simulink model "GesamtAblaufDiagramm_1"  (R2012b)
settings: Solver=FixedStepDiscrete  StartTime=0.0  StopTime=25  RelTol=1e-3
libraries: commutil2 x12, c280xlib x11, c2833xlib x8, idelinklib_tgtpref x2
(part 1 of 2)
settings Model: Creator=mit064  LastModifiedBy=Gelin Wang
settings DataIOCC: SaveOutput=off  SaveTime=off
settings OptimizationCC: OptimizeModelRefInitCode=on  LifeSpan=1
settings HardwareCC: ProdBitPerChar=16  ProdBitPerInt=16  ProdBitPerPointer=16  ProdLargestAtomicInteger=Integer  ProdIntDivRoundTo=Zero  ProdEndianess=LittleEndian  ProdWordSize=16  ProdHWDeviceType=Texas Instruments->C2000
settings RTWCC: SystemTargetFile=idelink_ert.tlc  GenerateMakefile=off  TemplateMakefile=none  Description=IDE Link ERT  ProcessScript=idelink_ert_make_rtw_hook
settings CodeAppCC: IgnoreCustomStorageClasses=off

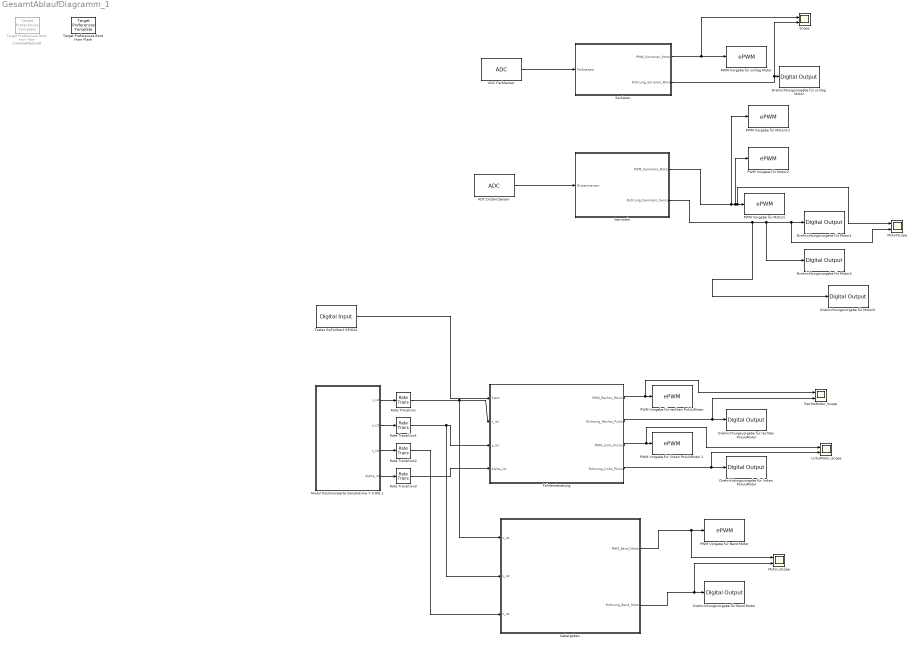
== system GesamtAblaufDiagramm_1 ==
  ADC DistanzSensor : c280xlib/ADC  useModule=A  useMode=Sequential  sourceSOC=Software  sourceSOC1=Software  sourceSOC2=ePWMxB  xint2_ADCSOC=31  Ts=0.001  dType=uint16  postInterrupt=off  numConversionsSingle=1  numConversionsDouble=1  conv0=ADCINA0  conv1=ADCINA1  conv2=ADCINA2  conv3=ADCINA3  conv4=ADCINA4  conv5=ADCINA5  conv6=ADCINA6  conv7=ADCINA7  conv8=ADCINB0  conv9=ADCINB1  conv10=ADCINB2  conv11=ADCINB3  conv12=ADCINB4  conv13=ADCINB5  conv14=ADCINB6  conv15=ADCINB7  convAB0=ADCINA0 and ADCINB0  convAB1=ADCINA1 and ADCINB1  convAB2=ADCINA2 and ADCINB2  convAB3=ADCINA3 and ADCINB3  convAB4=ADCINA4 and ADCINB4  convAB5=ADCINA5 and ADCINB5  convAB6=ADCINA6 and ADCINB6  convAB7=ADCINA7 and ADCINB7  convA0=ADCINA0  convA1=ADCINA1  convA2=ADCINA2  convA3=ADCINA3  convA4=ADCINA4  convA5=ADCINA5  convA6=ADCINA6  convA7=ADCINA7  convB0=ADCINB0  convB1=ADCINB1  convB2=ADCINB2  convB3=ADCINB3  convB4=ADCINB4  convB5=ADCINB5  convB6=ADCINB6  convB7=ADCINB7  c28xmultiPort=off  endma=off  chdma=1
  ADC FarbSensor : c280xlib/ADC  useModule=A  useMode=Sequential  sourceSOC=Software  sourceSOC1=Software  sourceSOC2=ePWMxB  xint2_ADCSOC=31  Ts=0.001  dType=uint16  postInterrupt=off  numConversionsSingle=1  numConversionsDouble=1  conv0=ADCINA0  conv1=ADCINA1  conv2=ADCINA2  conv3=ADCINA3  conv4=ADCINA4  conv5=ADCINA5  conv6=ADCINA6  conv7=ADCINA7  conv8=ADCINB0  conv9=ADCINB1  conv10=ADCINB2  conv11=ADCINB3  conv12=ADCINB4  conv13=ADCINB5  conv14=ADCINB6  conv15=ADCINB7  convAB0=ADCINA0 and ADCINB0  convAB1=ADCINA1 and ADCINB1  convAB2=ADCINA2 and ADCINB2  convAB3=ADCINA3 and ADCINB3  convAB4=ADCINA4 and ADCINB4  convAB5=ADCINA5 and ADCINB5  convAB6=ADCINA6 and ADCINB6  convAB7=ADCINA7 and ADCINB7  convA0=ADCINA0  convA1=ADCINA1  convA2=ADCINA2  convA3=ADCINA3  convA4=ADCINA4  convA5=ADCINA5  convA6=ADCINA6  convA7=ADCINA7  convB0=ADCINB0  convB1=ADCINB1  convB2=ADCINB2  convB3=ADCINB3  convB4=ADCINB4  convB5=ADCINB5  convB6=ADCINB6  convB7=ADCINB7  c28xmultiPort=off  endma=off  chdma=1
  Drehrichtungsvorgabe für Band Motor : c2833xlib/Digital Output  GPIO_Number=GPIO16~GPIO23  GPIO_Bit0=off  GPIO_BIT0_Toggle=off  GPIO_Bit1=off  GPIO_BIT1_Toggle=off  GPIO_Bit2=off  GPIO_BIT2_Toggle=off  GPIO_Bit3=off  GPIO_BIT3_Toggle=off  GPIO_Bit4=off  GPIO_BIT4_Toggle=off  GPIO_Bit5=on  GPIO_BIT5_Toggle=off  GPIO_Bit6=off  GPIO_BIT6_Toggle=off  GPIO_Bit7=off  GPIO_BIT7_Toggle=off
  Drehrichtungsvorgabe für Motor1 : c2833xlib/Digital Output  GPIO_Number=GPIO16~GPIO23  GPIO_Bit0=off  GPIO_BIT0_Toggle=off  GPIO_Bit1=off  GPIO_BIT1_Toggle=off  GPIO_Bit2=off  GPIO_BIT2_Toggle=off  GPIO_Bit3=off  GPIO_BIT3_Toggle=off  GPIO_Bit4=off  GPIO_BIT4_Toggle=off  GPIO_Bit5=on  GPIO_BIT5_Toggle=off  GPIO_Bit6=off  GPIO_BIT6_Toggle=off  GPIO_Bit7=off  GPIO_BIT7_Toggle=off
  Drehrichtungsvorgabe für Motor2 : c2833xlib/Digital Output  GPIO_Number=GPIO16~GPIO23  GPIO_Bit0=off  GPIO_BIT0_Toggle=off  GPIO_Bit1=off  GPIO_BIT1_Toggle=off  GPIO_Bit2=off  GPIO_BIT2_Toggle=off  GPIO_Bit3=off  GPIO_BIT3_Toggle=off  GPIO_Bit4=off  GPIO_BIT4_Toggle=off  GPIO_Bit5=on  GPIO_BIT5_Toggle=off  GPIO_Bit6=off  GPIO_BIT6_Toggle=off  GPIO_Bit7=off  GPIO_BIT7_Toggle=off
  Drehrichtungsvorgabe für Motor3 : c2833xlib/Digital Output  GPIO_Number=GPIO16~GPIO23  GPIO_Bit0=off  GPIO_BIT0_Toggle=off  GPIO_Bit1=off  GPIO_BIT1_Toggle=off  GPIO_Bit2=off  GPIO_BIT2_Toggle=off  GPIO_Bit3=off  GPIO_BIT3_Toggle=off  GPIO_Bit4=off  GPIO_BIT4_Toggle=off  GPIO_Bit5=on  GPIO_BIT5_Toggle=off  GPIO_Bit6=off  GPIO_BIT6_Toggle=off  GPIO_Bit7=off  GPIO_BIT7_Toggle=off
  Drehrichtungsvorgabe für linken PoluluMotor : c2833xlib/Digital Output  GPIO_Number=GPIO16~GPIO23  GPIO_Bit0=off  GPIO_BIT0_Toggle=off  GPIO_Bit1=off  GPIO_BIT1_Toggle=off  GPIO_Bit2=off  GPIO_BIT2_Toggle=off  GPIO_Bit3=off  GPIO_BIT3_Toggle=off  GPIO_Bit4=off  GPIO_BIT4_Toggle=off  GPIO_Bit5=on  GPIO_BIT5_Toggle=off  GPIO_Bit6=off  GPIO_BIT6_Toggle=off  GPIO_Bit7=off  GPIO_BIT7_Toggle=off
  Drehrichtungsvorgabe für rechten PoluluMotor : c2833xlib/Digital Output  GPIO_Number=GPIO16~GPIO23  GPIO_Bit0=off  GPIO_BIT0_Toggle=off  GPIO_Bit1=off  GPIO_BIT1_Toggle=off  GPIO_Bit2=off  GPIO_BIT2_Toggle=off  GPIO_Bit3=off  GPIO_BIT3_Toggle=off  GPIO_Bit4=off  GPIO_BIT4_Toggle=off  GPIO_Bit5=on  GPIO_BIT5_Toggle=off  GPIO_Bit6=off  GPIO_BIT6_Toggle=off  GPIO_Bit7=off  GPIO_BIT7_Toggle=off
  Drehrichtungsvorgabe für schlag Motor : c2833xlib/Digital Output  GPIO_Number=GPIO16~GPIO23  GPIO_Bit0=off  GPIO_BIT0_Toggle=off  GPIO_Bit1=off  GPIO_BIT1_Toggle=off  GPIO_Bit2=off  GPIO_BIT2_Toggle=off  GPIO_Bit3=off  GPIO_BIT3_Toggle=off  GPIO_Bit4=off  GPIO_BIT4_Toggle=off  GPIO_Bit5=on  GPIO_BIT5_Toggle=off  GPIO_Bit6=off  GPIO_BIT6_Toggle=off  GPIO_Bit7=off  GPIO_BIT7_Toggle=off
  "Fahransteuerung " : Subsystem
  LinksMotor_Scope : Scope  NumInputPorts=2
      settings: YMin=-5~-5  YMax=5~5  SaveName=ScopeData3
  Modul Positionswerte Sampletime = 0.001 s : Subsystem
  MotorScope : Scope  NumInputPorts=2
      settings: YMin=-5~-5  YMax=100~5  SaveName=ScopeData4
  Motor_Scope : Scope  NumInputPorts=2
      settings: YMin=-5~-5  YMax=5~5
  "PWM Vorgabe für Band Motor " : c280xlib/ePWM  checkMode=off  useModule=ePWM2  periodUnits=Clock cycles  timerSource=Specify via dialog  timerPeriod_clk=64000  timerPeriod_sec=0.0001  countingMode=Up  synchronizationOption=Disable  synchronizationEnable=off  phaseActiveEnable=Disable  phaseDirection=Count down after sync  phaseActive=0  clockPrescale=1  HSclockPrescale=1  ePWMxAStatus=off  CMPAUnits=Clock cycles  CMPASource=Specify via dialog  CMPAValue_per=50  CMPAValue_clk=32000  ePWMxAactionLogic1=Do nothing  ePWMxAactionLogic2=Clear  ePWMxAactionLogic3=Set  ePWMxAactionLogic4=Do nothing  ePWMxAactionLogic5=Do nothing  ePWMxAactionLogic6=Do nothing  ePWMxALoadMode=Load on CTR=Zero  ePWMxACSFenable=off  ePWMxACSFvalue=Forcing Disable  ePWMxASFreload=Zero  enHRPWM=off  HRPWM_LoadMode=CTR=ZERO  HRPWM_CTLMode=Phase control mode  HRPWM_EDGMode=Both edge  enSFO=on  ePWMxBStatus=on  CMPBUnits=Percentages  CMPBSource=Input port  CMPBValue_per=0  CMPBValue_clk=32000  ePWMxBactionLogic1=Do nothing  ePWMxBactionLogic2=Set  ePWMxBactionLogic3=Do nothing  ePWMxBactionLogic4=Do nothing  ePWMxBactionLogic5=Clear  ePWMxBactionLogic6=Do nothing  ePWMxBLoadMode=Load on CTR=Zero  ePWMxBCSFenable=off  ePWMxBCSFvalue=Forcing Disable  ePWMxBSFreload=Zero  enableDBePWMxA=off  enableDBePWMxB=off  DBpolarity=AH  DBedgeDelay=Positive  DBSource_ePWMxA=ePWMxA  DBSource_ePWMxB=ePWMxA  DBperiodSource=Specify via dialog  REDperiod=0  FEDperiod=0  adcstartModuleA=off  adcrequestEventA=First event  adcstartEventA=CTR=Zero  adcstartModuleB=off  adcrequestEventB=First event  adcstartEventB=CTR=Zero  intEn=off  intPrd=First event  intSel=CTR=Zero  chopperEnable=off  chopperFrequency=1  chopperFirstwidth=1  chopperDuty=12.5%  tripZonesource=Specify via dialog  tzselOSHT1=off  tzselOSHT2=off  tzselOSHT3=off  tzselOSHT4=off  tzselOSHT5=off  tzselOSHT6=off  tzselCBC1=off  tzselCBC2=off  tzselCBC3=off  tzselCBC4=off  tzselCBC5=off  tzselCBC6=off  enTzOstIntr=off  enTzCbcIntr=off  ePWMxAforced=No action  ePWMxBforced=No action  timerPeriod=-1  ePWMxAValue=0  ePWMxBValue=0  tripZoneoption=OSHT
  "PWM Vorgabe für Motor1 " : c280xlib/ePWM  checkMode=off  useModule=ePWM2  periodUnits=Clock cycles  timerSource=Specify via dialog  timerPeriod_clk=64000  timerPeriod_sec=0.0001  countingMode=Up  synchronizationOption=Disable  synchronizationEnable=off  phaseActiveEnable=Disable  phaseDirection=Count down after sync  phaseActive=0  clockPrescale=1  HSclockPrescale=1  ePWMxAStatus=off  CMPAUnits=Clock cycles  CMPASource=Specify via dialog  CMPAValue_per=50  CMPAValue_clk=32000  ePWMxAactionLogic1=Do nothing  ePWMxAactionLogic2=Clear  ePWMxAactionLogic3=Set  ePWMxAactionLogic4=Do nothing  ePWMxAactionLogic5=Do nothing  ePWMxAactionLogic6=Do nothing  ePWMxALoadMode=Load on CTR=Zero  ePWMxACSFenable=off  ePWMxACSFvalue=Forcing Disable  ePWMxASFreload=Zero  enHRPWM=off  HRPWM_LoadMode=CTR=ZERO  HRPWM_CTLMode=Phase control mode  HRPWM_EDGMode=Both edge  enSFO=on  ePWMxBStatus=on  CMPBUnits=Percentages  CMPBSource=Input port  CMPBValue_per=0  CMPBValue_clk=32000  ePWMxBactionLogic1=Do nothing  ePWMxBactionLogic2=Set  ePWMxBactionLogic3=Do nothing  ePWMxBactionLogic4=Do nothing  ePWMxBactionLogic5=Clear  ePWMxBactionLogic6=Do nothing  ePWMxBLoadMode=Load on CTR=Zero  ePWMxBCSFenable=off  ePWMxBCSFvalue=Forcing Disable  ePWMxBSFreload=Zero  enableDBePWMxA=off  enableDBePWMxB=off  DBpolarity=AH  DBedgeDelay=Positive  DBSource_ePWMxA=ePWMxA  DBSource_ePWMxB=ePWMxA  DBperiodSource=Specify via dialog  REDperiod=0  FEDperiod=0  adcstartModuleA=off  adcrequestEventA=First event  adcstartEventA=CTR=Zero  adcstartModuleB=off  adcrequestEventB=First event  adcstartEventB=CTR=Zero  intEn=off  intPrd=First event  intSel=CTR=Zero  chopperEnable=off  chopperFrequency=1  chopperFirstwidth=1  chopperDuty=12.5%  tripZonesource=Specify via dialog  tzselOSHT1=off  tzselOSHT2=off  tzselOSHT3=off  tzselOSHT4=off  tzselOSHT5=off  tzselOSHT6=off  tzselCBC1=off  tzselCBC2=off  tzselCBC3=off  tzselCBC4=off  tzselCBC5=off  tzselCBC6=off  enTzOstIntr=off  enTzCbcIntr=off  ePWMxAforced=No action  ePWMxBforced=No action  timerPeriod=-1  ePWMxAValue=0  ePWMxBValue=0  tripZoneoption=OSHT
  "PWM Vorgabe für Motor2 " : c280xlib/ePWM  checkMode=off  useModule=ePWM2  periodUnits=Clock cycles  timerSource=Specify via dialog  timerPeriod_clk=64000  timerPeriod_sec=0.0001  countingMode=Up  synchronizationOption=Disable  synchronizationEnable=off  phaseActiveEnable=Disable  phaseDirection=Count down after sync  phaseActive=0  clockPrescale=1  HSclockPrescale=1  ePWMxAStatus=off  CMPAUnits=Clock cycles  CMPASource=Specify via dialog  CMPAValue_per=50  CMPAValue_clk=32000  ePWMxAactionLogic1=Do nothing  ePWMxAactionLogic2=Clear  ePWMxAactionLogic3=Set  ePWMxAactionLogic4=Do nothing  ePWMxAactionLogic5=Do nothing  ePWMxAactionLogic6=Do nothing  ePWMxALoadMode=Load on CTR=Zero  ePWMxACSFenable=off  ePWMxACSFvalue=Forcing Disable  ePWMxASFreload=Zero  enHRPWM=off  HRPWM_LoadMode=CTR=ZERO  HRPWM_CTLMode=Phase control mode  HRPWM_EDGMode=Both edge  enSFO=on  ePWMxBStatus=on  CMPBUnits=Percentages  CMPBSource=Input port  CMPBValue_per=0  CMPBValue_clk=32000  ePWMxBactionLogic1=Do nothing  ePWMxBactionLogic2=Set  ePWMxBactionLogic3=Do nothing  ePWMxBactionLogic4=Do nothing  ePWMxBactionLogic5=Clear  ePWMxBactionLogic6=Do nothing  ePWMxBLoadMode=Load on CTR=Zero  ePWMxBCSFenable=off  ePWMxBCSFvalue=Forcing Disable  ePWMxBSFreload=Zero  enableDBePWMxA=off  enableDBePWMxB=off  DBpolarity=AH  DBedgeDelay=Positive  DBSource_ePWMxA=ePWMxA  DBSource_ePWMxB=ePWMxA  DBperiodSource=Specify via dialog  REDperiod=0  FEDperiod=0  adcstartModuleA=off  adcrequestEventA=First event  adcstartEventA=CTR=Zero  adcstartModuleB=off  adcrequestEventB=First event  adcstartEventB=CTR=Zero  intEn=off  intPrd=First event  intSel=CTR=Zero  chopperEnable=off  chopperFrequency=1  chopperFirstwidth=1  chopperDuty=12.5%  tripZonesource=Specify via dialog  tzselOSHT1=off  tzselOSHT2=off  tzselOSHT3=off  tzselOSHT4=off  tzselOSHT5=off  tzselOSHT6=off  tzselCBC1=off  tzselCBC2=off  tzselCBC3=off  tzselCBC4=off  tzselCBC5=off  tzselCBC6=off  enTzOstIntr=off  enTzCbcIntr=off  ePWMxAforced=No action  ePWMxBforced=No action  timerPeriod=-1  ePWMxAValue=0  ePWMxBValue=0  tripZoneoption=OSHT
  PWM Vorgabe für Motor3 2 : c280xlib/ePWM  checkMode=off  useModule=ePWM2  periodUnits=Clock cycles  timerSource=Specify via dialog  timerPeriod_clk=64000  timerPeriod_sec=0.0001  countingMode=Up  synchronizationOption=Disable  synchronizationEnable=off  phaseActiveEnable=Disable  phaseDirection=Count down after sync  phaseActive=0  clockPrescale=1  HSclockPrescale=1  ePWMxAStatus=off  CMPAUnits=Clock cycles  CMPASource=Specify via dialog  CMPAValue_per=50  CMPAValue_clk=32000  ePWMxAactionLogic1=Do nothing  ePWMxAactionLogic2=Clear  ePWMxAactionLogic3=Set  ePWMxAactionLogic4=Do nothing  ePWMxAactionLogic5=Do nothing  ePWMxAactionLogic6=Do nothing  ePWMxALoadMode=Load on CTR=Zero  ePWMxACSFenable=off  ePWMxACSFvalue=Forcing Disable  ePWMxASFreload=Zero  enHRPWM=off  HRPWM_LoadMode=CTR=ZERO  HRPWM_CTLMode=Phase control mode  HRPWM_EDGMode=Both edge  enSFO=on  ePWMxBStatus=on  CMPBUnits=Percentages  CMPBSource=Input port  CMPBValue_per=0  CMPBValue_clk=32000  ePWMxBactionLogic1=Do nothing  ePWMxBactionLogic2=Set  ePWMxBactionLogic3=Do nothing  ePWMxBactionLogic4=Do nothing  ePWMxBactionLogic5=Clear  ePWMxBactionLogic6=Do nothing  ePWMxBLoadMode=Load on CTR=Zero  ePWMxBCSFenable=off  ePWMxBCSFvalue=Forcing Disable  ePWMxBSFreload=Zero  enableDBePWMxA=off  enableDBePWMxB=off  DBpolarity=AH  DBedgeDelay=Positive  DBSource_ePWMxA=ePWMxA  DBSource_ePWMxB=ePWMxA  DBperiodSource=Specify via dialog  REDperiod=0  FEDperiod=0  adcstartModuleA=off  adcrequestEventA=First event  adcstartEventA=CTR=Zero  adcstartModuleB=off  adcrequestEventB=First event  adcstartEventB=CTR=Zero  intEn=off  intPrd=First event  intSel=CTR=Zero  chopperEnable=off  chopperFrequency=1  chopperFirstwidth=1  chopperDuty=12.5%  tripZonesource=Specify via dialog  tzselOSHT1=off  tzselOSHT2=off  tzselOSHT3=off  tzselOSHT4=off  tzselOSHT5=off  tzselOSHT6=off  tzselCBC1=off  tzselCBC2=off  tzselCBC3=off  tzselCBC4=off  tzselCBC5=off  tzselCBC6=off  enTzOstIntr=off  enTzCbcIntr=off  ePWMxAforced=No action  ePWMxBforced=No action  timerPeriod=-1  ePWMxAValue=0  ePWMxBValue=0  tripZoneoption=OSHT
  PWM Vorgabe für linken PoluluMotor 1 : c280xlib/ePWM  checkMode=off  useModule=ePWM2  periodUnits=Clock cycles  timerSource=Specify via dialog  timerPeriod_clk=64000  timerPeriod_sec=0.0001  countingMode=Up  synchronizationOption=Disable  synchronizationEnable=off  phaseActiveEnable=Disable  phaseDirection=Count down after sync  phaseActive=0  clockPrescale=1  HSclockPrescale=1  ePWMxAStatus=off  CMPAUnits=Clock cycles  CMPASource=Specify via dialog  CMPAValue_per=50  CMPAValue_clk=32000  ePWMxAactionLogic1=Do nothing  ePWMxAactionLogic2=Clear  ePWMxAactionLogic3=Set  ePWMxAactionLogic4=Do nothing  ePWMxAactionLogic5=Do nothing  ePWMxAactionLogic6=Do nothing  ePWMxALoadMode=Load on CTR=Zero  ePWMxACSFenable=off  ePWMxACSFvalue=Forcing Disable  ePWMxASFreload=Zero  enHRPWM=off  HRPWM_LoadMode=CTR=ZERO  HRPWM_CTLMode=Phase control mode  HRPWM_EDGMode=Both edge  enSFO=on  ePWMxBStatus=on  CMPBUnits=Percentages  CMPBSource=Input port  CMPBValue_per=0  CMPBValue_clk=32000  ePWMxBactionLogic1=Do nothing  ePWMxBactionLogic2=Set  ePWMxBactionLogic3=Do nothing  ePWMxBactionLogic4=Do nothing  ePWMxBactionLogic5=Clear  ePWMxBactionLogic6=Do nothing  ePWMxBLoadMode=Load on CTR=Zero  ePWMxBCSFenable=off  ePWMxBCSFvalue=Forcing Disable  ePWMxBSFreload=Zero  enableDBePWMxA=off  enableDBePWMxB=off  DBpolarity=AH  DBedgeDelay=Positive  DBSource_ePWMxA=ePWMxA  DBSource_ePWMxB=ePWMxA  DBperiodSource=Specify via dialog  REDperiod=0  FEDperiod=0  adcstartModuleA=off  adcrequestEventA=First event  adcstartEventA=CTR=Zero  adcstartModuleB=off  adcrequestEventB=First event  adcstartEventB=CTR=Zero  intEn=off  intPrd=First event  intSel=CTR=Zero  chopperEnable=off  chopperFrequency=1  chopperFirstwidth=1  chopperDuty=12.5%  tripZonesource=Specify via dialog  tzselOSHT1=off  tzselOSHT2=off  tzselOSHT3=off  tzselOSHT4=off  tzselOSHT5=off  tzselOSHT6=off  tzselCBC1=off  tzselCBC2=off  tzselCBC3=off  tzselCBC4=off  tzselCBC5=off  tzselCBC6=off  enTzOstIntr=off  enTzCbcIntr=off  ePWMxAforced=No action  ePWMxBforced=No action  timerPeriod=-1  ePWMxAValue=0  ePWMxBValue=0  tripZoneoption=OSHT
  "PWM Vorgabe für rechten PoluluMotor " : c280xlib/ePWM  checkMode=off  useModule=ePWM2  periodUnits=Clock cycles  timerSource=Specify via dialog  timerPeriod_clk=64000  timerPeriod_sec=0.0001  countingMode=Up  synchronizationOption=Disable  synchronizationEnable=off  phaseActiveEnable=Disable  phaseDirection=Count down after sync  phaseActive=0  clockPrescale=1  HSclockPrescale=1  ePWMxAStatus=off  CMPAUnits=Clock cycles  CMPASource=Specify via dialog  CMPAValue_per=50  CMPAValue_clk=32000  ePWMxAactionLogic1=Do nothing  ePWMxAactionLogic2=Clear  ePWMxAactionLogic3=Set  ePWMxAactionLogic4=Do nothing  ePWMxAactionLogic5=Do nothing  ePWMxAactionLogic6=Do nothing  ePWMxALoadMode=Load on CTR=Zero  ePWMxACSFenable=off  ePWMxACSFvalue=Forcing Disable  ePWMxASFreload=Zero  enHRPWM=off  HRPWM_LoadMode=CTR=ZERO  HRPWM_CTLMode=Phase control mode  HRPWM_EDGMode=Both edge  enSFO=on  ePWMxBStatus=on  CMPBUnits=Percentages  CMPBSource=Input port  CMPBValue_per=0  CMPBValue_clk=32000  ePWMxBactionLogic1=Do nothing  ePWMxBactionLogic2=Set  ePWMxBactionLogic3=Do nothing  ePWMxBactionLogic4=Do nothing  ePWMxBactionLogic5=Clear  ePWMxBactionLogic6=Do nothing  ePWMxBLoadMode=Load on CTR=Zero  ePWMxBCSFenable=off  ePWMxBCSFvalue=Forcing Disable  ePWMxBSFreload=Zero  enableDBePWMxA=off  enableDBePWMxB=off  DBpolarity=AH  DBedgeDelay=Positive  DBSource_ePWMxA=ePWMxA  DBSource_ePWMxB=ePWMxA  DBperiodSource=Specify via dialog  REDperiod=0  FEDperiod=0  adcstartModuleA=off  adcrequestEventA=First event  adcstartEventA=CTR=Zero  adcstartModuleB=off  adcrequestEventB=First event  adcstartEventB=CTR=Zero  intEn=off  intPrd=First event  intSel=CTR=Zero  chopperEnable=off  chopperFrequency=1  chopperFirstwidth=1  chopperDuty=12.5%  tripZonesource=Specify via dialog  tzselOSHT1=off  tzselOSHT2=off  tzselOSHT3=off  tzselOSHT4=off  tzselOSHT5=off  tzselOSHT6=off  tzselCBC1=off  tzselCBC2=off  tzselCBC3=off  tzselCBC4=off  tzselCBC5=off  tzselCBC6=off  enTzOstIntr=off  enTzCbcIntr=off  ePWMxAforced=No action  ePWMxBforced=No action  timerPeriod=-1  ePWMxAValue=0  ePWMxBValue=0  tripZoneoption=OSHT
  "PWM Vorgabe für schlag Motor " : c280xlib/ePWM  checkMode=off  useModule=ePWM2  periodUnits=Clock cycles  timerSource=Specify via dialog  timerPeriod_clk=64000  timerPeriod_sec=0.0001  countingMode=Up  synchronizationOption=Disable  synchronizationEnable=off  phaseActiveEnable=Disable  phaseDirection=Count down after sync  phaseActive=0  clockPrescale=1  HSclockPrescale=1  ePWMxAStatus=off  CMPAUnits=Clock cycles  CMPASource=Specify via dialog  CMPAValue_per=50  CMPAValue_clk=32000  ePWMxAactionLogic1=Do nothing  ePWMxAactionLogic2=Clear  ePWMxAactionLogic3=Set  ePWMxAactionLogic4=Do nothing  ePWMxAactionLogic5=Do nothing  ePWMxAactionLogic6=Do nothing  ePWMxALoadMode=Load on CTR=Zero  ePWMxACSFenable=off  ePWMxACSFvalue=Forcing Disable  ePWMxASFreload=Zero  enHRPWM=off  HRPWM_LoadMode=CTR=ZERO  HRPWM_CTLMode=Phase control mode  HRPWM_EDGMode=Both edge  enSFO=on  ePWMxBStatus=on  CMPBUnits=Percentages  CMPBSource=Input port  CMPBValue_per=0  CMPBValue_clk=32000  ePWMxBactionLogic1=Do nothing  ePWMxBactionLogic2=Set  ePWMxBactionLogic3=Do nothing  ePWMxBactionLogic4=Do nothing  ePWMxBactionLogic5=Clear  ePWMxBactionLogic6=Do nothing  ePWMxBLoadMode=Load on CTR=Zero  ePWMxBCSFenable=off  ePWMxBCSFvalue=Forcing Disable  ePWMxBSFreload=Zero  enableDBePWMxA=off  enableDBePWMxB=off  DBpolarity=AH  DBedgeDelay=Positive  DBSource_ePWMxA=ePWMxA  DBSource_ePWMxB=ePWMxA  DBperiodSource=Specify via dialog  REDperiod=0  FEDperiod=0  adcstartModuleA=off  adcrequestEventA=First event  adcstartEventA=CTR=Zero  adcstartModuleB=off  adcrequestEventB=First event  adcstartEventB=CTR=Zero  intEn=off  intPrd=First event  intSel=CTR=Zero  chopperEnable=off  chopperFrequency=1  chopperFirstwidth=1  chopperDuty=12.5%  tripZonesource=Specify via dialog  tzselOSHT1=off  tzselOSHT2=off  tzselOSHT3=off  tzselOSHT4=off  tzselOSHT5=off  tzselOSHT6=off  tzselCBC1=off  tzselCBC2=off  tzselCBC3=off  tzselCBC4=off  tzselCBC5=off  tzselCBC6=off  enTzOstIntr=off  enTzCbcIntr=off  ePWMxAforced=No action  ePWMxBforced=No action  timerPeriod=-1  ePWMxAValue=0  ePWMxBValue=0  tripZoneoption=OSHT
  Rate Transition{,1..3} (4 alike) : RateTransition  OutPortSampleTime=0.01
  RechtsMotor_Scope : Scope  NumInputPorts=2
      settings: YMin=-5~-5  YMax=5~5  SaveName=ScopeData2
  Sammeln : Subsystem
  Scope : Scope  NumInputPorts=2
      settings: YMin=-5~-5  YMax=5~5
  Sortieren : Subsystem
  Target Preferences Boot from Flash : idelinklib_tgtpref/Target Preferences Template  Tag=ccslinktgtpref_ccsv4  library=off
  Target Preferences Boot from Ram : idelinklib_tgtpref/Target Preferences Template  Tag=ccslinktgtpref_ccsv4  Commented=on  library=off
  Taster GoForStart GPIO24 : c2833xlib/Digital Input  GPIO_Number=GPIO24~GPIO31  GPIO_Bit0=on  GPIO_Bit1=off  GPIO_Bit2=off  GPIO_Bit3=off  GPIO_Bit4=off  GPIO_Bit5=off  GPIO_Bit6=off  GPIO_Bit7=off  sampleTime=0.001  dataType=auto  GPIO_Bit0_Qualification=Sync to SYSCLKOUT  GPIO_Bit1_Qualification=Sync to SYSCLKOUT  GPIO_Bit2_Qualification=Sync to SYSCLKOUT  GPIO_Bit3_Qualification=Sync to SYSCLKOUT  GPIO_Bit4_Qualification=Sync to SYSCLKOUT  GPIO_Bit5_Qualification=Sync to SYSCLKOUT  GPIO_Bit6_Qualification=Sync to SYSCLKOUT  GPIO_Bit7_Qualification=Sync to SYSCLKOUT  Qualification_Period=-1
  Uebergeben : Subsystem
  wires:
  Modul Positionswerte Sampletime = 0.001 s/1(x_ist) -> Rate Transition/1
  Modul Positionswerte Sampletime = 0.001 s/4(alpha_ist) -> Rate Transition3/1
  Modul Positionswerte Sampletime = 0.001 s/3(z_ist) -> Rate Transition2/1
  Modul Positionswerte Sampletime = 0.001 s/2(y_ist) -> Rate Transition1/1
  Rate Transition/1 -> Uebergeben/1(x_ist), "Fahransteuerung "/2(x_ist)
  Rate Transition1/1 -> Uebergeben/2(y_ist), "Fahransteuerung "/3(y_ist)
  Rate Transition3/1 -> "Fahransteuerung "/4(alpha_ist)
  "Fahransteuerung "/1(PWM_Rechts_Polulu) -> RechtsMotor_Scope/1, "PWM Vorgabe für rechten PoluluMotor "/1
  "Fahransteuerung "/2(Richtung_Rechts_Pulolo) -> RechtsMotor_Scope/2, Drehrichtungsvorgabe für rechten PoluluMotor/1
  "Fahransteuerung "/3(PWM_Links_Polulu) -> LinksMotor_Scope/1, PWM Vorgabe für linken PoluluMotor 1/1
  "Fahransteuerung "/4(Richtung_Links_Polulu) -> LinksMotor_Scope/2, Drehrichtungsvorgabe für linken PoluluMotor/1
  Rate Transition2/1 -> Uebergeben/3(z_ist)
  Uebergeben/1(PWM_Band_Motor) -> Motor_Scope/1, "PWM Vorgabe für Band Motor "/1
  Uebergeben/2(Richtung_Band_Motor) -> Motor_Scope/2, Drehrichtungsvorgabe für Band Motor/1
  ADC DistanzSensor/1 -> Sammeln/1(Distanzsensor)
  ADC FarbSensor/1 -> Sortieren/1(Farbsensor)
  Sortieren/2(Richtung_Sorieren_Motor) -> Scope/2, Drehrichtungsvorgabe für schlag Motor/1
  Sortieren/1(PMW_Sortieren_Motor) -> Scope/1, "PWM Vorgabe für schlag Motor "/1
  Sammeln/2(Richtung_Sammeln_Sensor) -> Drehrichtungsvorgabe für Motor3/1, Drehrichtungsvorgabe für Motor2/1, MotorScope/2, Drehrichtungsvorgabe für Motor1/1
  Sammeln/1(PWM_Sammeln_Motor) -> PWM Vorgabe für Motor3 2/1, "PWM Vorgabe für Motor2 "/1, MotorScope/1, "PWM Vorgabe für Motor1 "/1
  Taster GoForStart GPIO24/1 -> "Fahransteuerung "/1(Start)

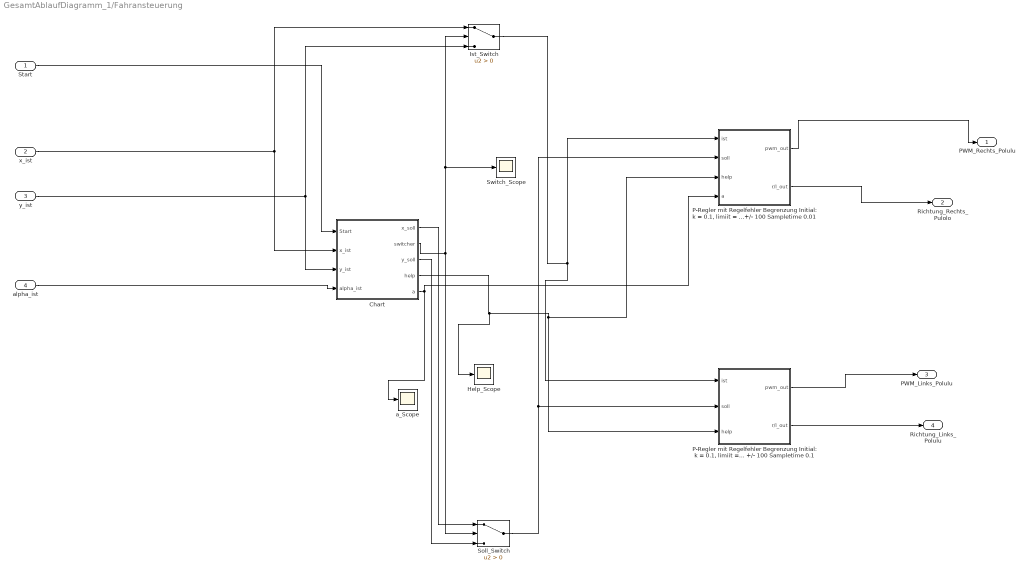
== system GesamtAblaufDiagramm_1/Fahransteuerung  ==
  Start : Inport
  x_ist : Inport  Port=2
  y_ist : Inport  Port=3
  alpha_ist : Inport  Port=4
  Chart : Stateflow chart  TreatAsAtomicUnit=on
  Help_Scope : Scope
      settings: SaveName=ScopeData5
  Ist_Switch : Switch  Criteria=u2 > Threshold
  "P-Regler mit Regelfehler Begrenzung Initial: k = 0.1, limiit = +/- 100 Sampletime 0.01" : Subsystem
  "P-Regler mit Regelfehler Begrenzung Initial: k = 0.1, limiit = +/- 100 Sampletime 0.1" : Subsystem
  Soll_Switch : Switch  Criteria=u2 > Threshold
  Switch_Scope : Scope
      settings: SaveName=ScopeData6
  a_Scope : Scope
      settings: SaveName=ScopeData7
  PWM_Rechts_Polulu : Outport
  Richtung_Rechts_Pulolo : Outport  Port=2
  PWM_Links_Polulu : Outport  Port=3
  Richtung_Links_Polulu : Outport  Port=4
  wires:
  "P-Regler mit Regelfehler Begrenzung Initial: k = 0.1, limiit = +/- 100 Sampletime 0.01"/2(r/l_out) -> Richtung_Rechts_Pulolo/1
  "P-Regler mit Regelfehler Begrenzung Initial: k = 0.1, limiit = +/- 100 Sampletime 0.01"/1(pwm_out) -> PWM_Rechts_Polulu/1
  Ist_Switch/1 -> "P-Regler mit Regelfehler Begrenzung Initial: k = 0.1, limiit = +/- 100 Sampletime 0.1"/1(ist), "P-Regler mit Regelfehler Begrenzung Initial: k = 0.1, limiit = +/- 100 Sampletime 0.01"/1(ist)
  Soll_Switch/1 -> "P-Regler mit Regelfehler Begrenzung Initial: k = 0.1, limiit = +/- 100 Sampletime 0.01"/2(soll), "P-Regler mit Regelfehler Begrenzung Initial: k = 0.1, limiit = +/- 100 Sampletime 0.1"/2(soll)
  Chart/2(switcher) -> Soll_Switch/2, Switch_Scope/1, Ist_Switch/2
  Chart/1(x_soll) -> Soll_Switch/1
  Chart/3(y_soll) -> Soll_Switch/3
  Chart/4(help) -> Help_Scope/1, "P-Regler mit Regelfehler Begrenzung Initial: k = 0.1, limiit = +/- 100 Sampletime 0.01"/3(help), "P-Regler mit Regelfehler Begrenzung Initial: k = 0.1, limiit = +/- 100 Sampletime 0.1"/3(help)
  x_ist/1 -> Chart/2(x_ist), Ist_Switch/1
  y_ist/1 -> Chart/3(y_ist), Ist_Switch/3
  alpha_ist/1 -> Chart/4(alpha_ist)
  "P-Regler mit Regelfehler Begrenzung Initial: k = 0.1, limiit = +/- 100 Sampletime 0.1"/1(pwm_out) -> PWM_Links_Polulu/1
  "P-Regler mit Regelfehler Begrenzung Initial: k = 0.1, limiit = +/- 100 Sampletime 0.1"/2(r/l_out) -> Richtung_Links_Polulu/1
  Chart/5(a) -> a_Scope/1, "P-Regler mit Regelfehler Begrenzung Initial: k = 0.1, limiit = +/- 100 Sampletime 0.01"/4(a)
  Start/1 -> Chart/1(Start)

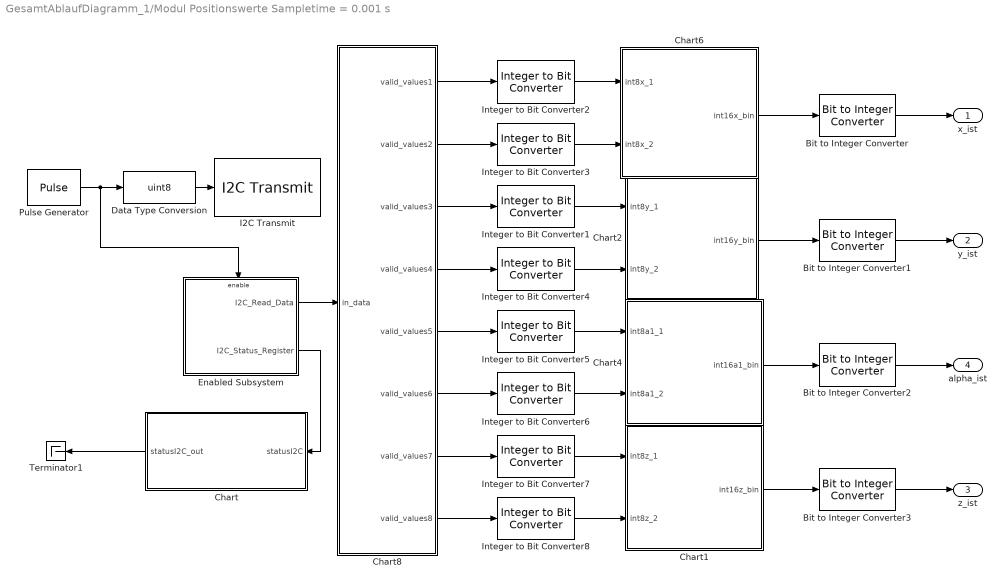
== system GesamtAblaufDiagramm_1/Modul Positionswerte Sampletime = 0.001 s ==
  Bit to Integer Converter{,1..3} (4 alike) : commutil2/Bit to Integer Converter  nbits=16  bitOrder=MSB first  signedOutputValues=Signed  outDtype=Inherit via internal rule  outDtypeSigned=Inherit via internal rule
  Chart : Stateflow chart  TreatAsAtomicUnit=on
  Chart1 : Stateflow chart  TreatAsAtomicUnit=on
  Chart2 : Stateflow chart  TreatAsAtomicUnit=on
  Chart4 : Stateflow chart  TreatAsAtomicUnit=on
  Chart6 : Stateflow chart  TreatAsAtomicUnit=on
  Chart8 : Stateflow chart  TreatAsAtomicUnit=on
  Data Type Conversion : DataTypeConversion  OutDataTypeStr=uint8
  Enabled Subsystem : Subsystem  TreatAsAtomicUnit=on
  I2C Transmit : c280xlib/I2C Transmit  addrFormat=7-Bit addressing  saSource=Specify via dialog  SAR=80  bitCount=8  STP=off  RM=off  STR=off
  Integer to Bit Converter{1..8} (8 alike) : commutil2/Integer to Bit Converter  nbits=8  signedInputValues=Unsigned  bitOrder=MSB first  outDtype=uint8
  Pulse Generator : DiscretePulseGenerator  Period=250  PulseWidth=249  SampleTime=0.001
  Terminator1 : Terminator
  x_ist : Outport
  y_ist : Outport  Port=2
  z_ist : Outport  Port=3
  alpha_ist : Outport  Port=4
  wires:
  Chart8/5(valid_values5) -> Integer to Bit Converter5/1
  Chart8/2(valid_values2) -> Integer to Bit Converter3/1
  Chart8/4(valid_values4) -> Integer to Bit Converter4/1
  Chart2/1(int16y_bin) -> Bit to Integer Converter1/1
  Chart8/1(valid_values1) -> Integer to Bit Converter2/1
  Chart8/3(valid_values3) -> Integer to Bit Converter1/1
  Integer to Bit Converter3/1 -> Chart6/2(int8x_2)
  Chart6/1(int16x_bin) -> Bit to Integer Converter/1
  Integer to Bit Converter1/1 -> Chart2/1(int8y_1)
  Integer to Bit Converter2/1 -> Chart6/1(int8x_1)
  Integer to Bit Converter4/1 -> Chart2/2(int8y_2)
  Bit to Integer Converter1/1 -> y_ist/1
  Integer to Bit Converter5/1 -> Chart4/1(int8a1_1)
  Integer to Bit Converter6/1 -> Chart4/2(int8a1_2)
  Bit to Integer Converter/1 -> x_ist/1
  Bit to Integer Converter2/1 -> alpha_ist/1
  Chart8/6(valid_values6) -> Integer to Bit Converter6/1
  Chart4/1(int16a1_bin) -> Bit to Integer Converter2/1
  Chart1/1(int16z_bin) -> Bit to Integer Converter3/1
  Enabled Subsystem/1(I2C_Read_Data) -> Chart8/1(in_data)
  Bit to Integer Converter3/1 -> z_ist/1
  Chart8/8(valid_values8) -> Integer to Bit Converter8/1
  Chart8/7(valid_values7) -> Integer to Bit Converter7/1
  Integer to Bit Converter8/1 -> Chart1/2(int8z_2)
  Integer to Bit Converter7/1 -> Chart1/1(int8z_1)
  Enabled Subsystem/2(I2C_Status_Register) -> Chart/1(statusI2C)
  Chart/1(statusI2C_out) -> Terminator1/1
  Pulse Generator/1 -> Enabled Subsystem/Enable, Data Type Conversion/1
  Data Type Conversion/1 -> I2C Transmit/1

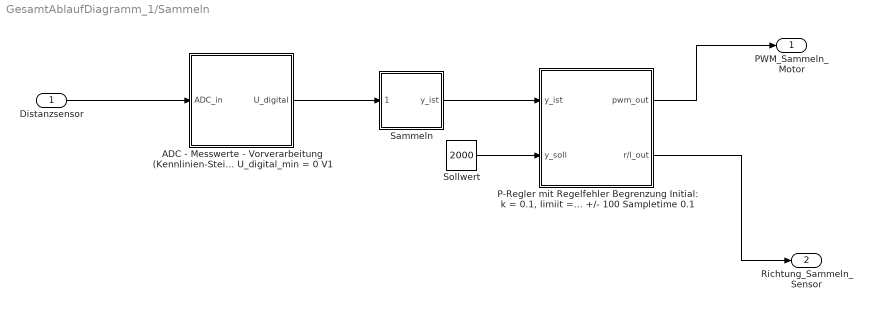
== system GesamtAblaufDiagramm_1/Sammeln ==
  Distanzsensor : Inport
  ADC - Messwerte - Vorverarbeitung (Kennlinien-Steigung und Offset-Kompensation) U_digital = (ADC_in - Offset) * 3.546 V / 4096 mit U_digital_max = 3.546 V U_digital_min = 0 V1 : Subsystem
  "P-Regler mit Regelfehler Begrenzung Initial: k = 0.1, limiit = +/- 100 Sampletime 0.1" : Subsystem
  Sammeln : Stateflow chart  TreatAsAtomicUnit=on
  Sollwert : Constant  Value=2000
  PWM_Sammeln_Motor : Outport
  Richtung_Sammeln_Sensor : Outport  Port=2
  wires:
  Sollwert/1 -> "P-Regler mit Regelfehler Begrenzung Initial: k = 0.1, limiit = +/- 100 Sampletime 0.1"/2(y_soll)
  Distanzsensor/1 -> ADC - Messwerte - Vorverarbeitung (Kennlinien-Steigung und Offset-Kompensation) U_digital = (ADC_in - Offset) * 3.546 V / 4096 mit U_digital_max = 3.546 V U_digital_min = 0 V1/1(ADC_in)
  Sammeln/1(y_ist) -> "P-Regler mit Regelfehler Begrenzung Initial: k = 0.1, limiit = +/- 100 Sampletime 0.1"/1(y_ist)
  ADC - Messwerte - Vorverarbeitung (Kennlinien-Steigung und Offset-Kompensation) U_digital = (ADC_in - Offset) * 3.546 V / 4096 mit U_digital_max = 3.546 V U_digital_min = 0 V1/1(U_digital) -> Sammeln/1(U_digital)
  "P-Regler mit Regelfehler Begrenzung Initial: k = 0.1, limiit = +/- 100 Sampletime 0.1"/1(pwm_out) -> PWM_Sammeln_Motor/1
  "P-Regler mit Regelfehler Begrenzung Initial: k = 0.1, limiit = +/- 100 Sampletime 0.1"/2(r/l_out) -> Richtung_Sammeln_Sensor/1

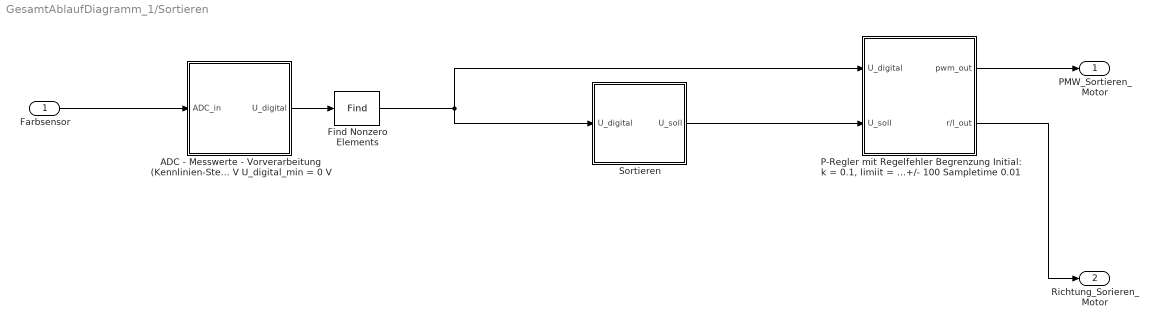
== system GesamtAblaufDiagramm_1/Sortieren ==
  Farbsensor : Inport
  ADC - Messwerte - Vorverarbeitung (Kennlinien-Steigung und Offset-Kompensation) U_digital = (ADC_in - Offset) * 3.546 V / 4096 mit U_digital_max = 3.546 V U_digital_min = 0 V : Subsystem
  Find Nonzero Elements : Find  NumberOfInputDimensions=3  IndexMode=Zero-based
  "P-Regler mit Regelfehler Begrenzung Initial: k = 0.1, limiit = +/- 100 Sampletime 0.01" : Subsystem
  Sortieren : Stateflow chart  TreatAsAtomicUnit=on
  PMW_Sortieren_Motor : Outport
  Richtung_Sorieren_Motor : Outport  Port=2
  wires:
  Farbsensor/1 -> ADC - Messwerte - Vorverarbeitung (Kennlinien-Steigung und Offset-Kompensation) U_digital = (ADC_in - Offset) * 3.546 V / 4096 mit U_digital_max = 3.546 V U_digital_min = 0 V/1(ADC_in)
  ADC - Messwerte - Vorverarbeitung (Kennlinien-Steigung und Offset-Kompensation) U_digital = (ADC_in - Offset) * 3.546 V / 4096 mit U_digital_max = 3.546 V U_digital_min = 0 V/1(U_digital) -> Find Nonzero Elements/1
  Find Nonzero Elements/1 -> Sortieren/1(U_digital), "P-Regler mit Regelfehler Begrenzung Initial: k = 0.1, limiit = +/- 100 Sampletime 0.01"/1(U_digital)
  Sortieren/1(U_soll) -> "P-Regler mit Regelfehler Begrenzung Initial: k = 0.1, limiit = +/- 100 Sampletime 0.01"/2(U_soll)
  "P-Regler mit Regelfehler Begrenzung Initial: k = 0.1, limiit = +/- 100 Sampletime 0.01"/1(pwm_out) -> PMW_Sortieren_Motor/1
  "P-Regler mit Regelfehler Begrenzung Initial: k = 0.1, limiit = +/- 100 Sampletime 0.01"/2(r/l_out) -> Richtung_Sorieren_Motor/1

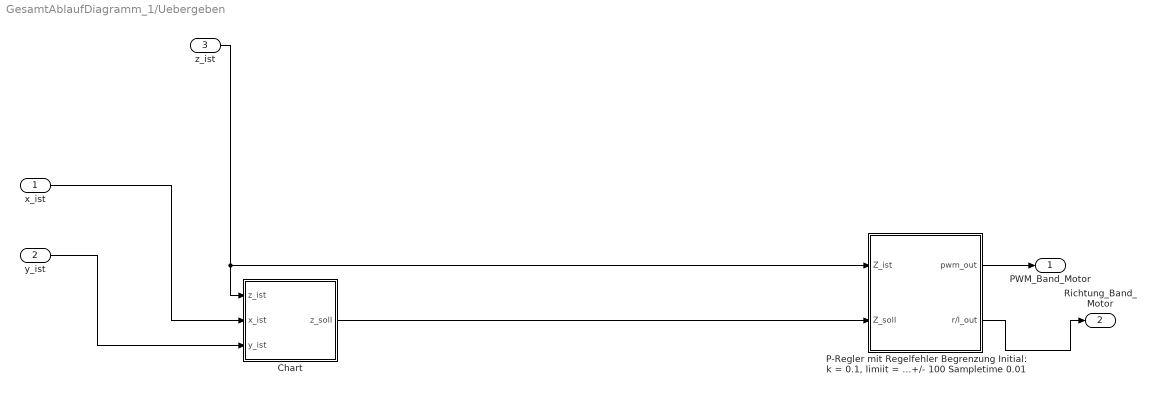
== system GesamtAblaufDiagramm_1/Uebergeben ==
  x_ist : Inport
  y_ist : Inport  Port=2
  z_ist : Inport  Port=3
  Chart : Stateflow chart  TreatAsAtomicUnit=on
  "P-Regler mit Regelfehler Begrenzung Initial: k = 0.1, limiit = +/- 100 Sampletime 0.01" : Subsystem
  PWM_Band_Motor : Outport
  Richtung_Band_Motor : Outport  Port=2
  wires:
  "P-Regler mit Regelfehler Begrenzung Initial: k = 0.1, limiit = +/- 100 Sampletime 0.01"/2(r/l_out) -> Richtung_Band_Motor/1
  "P-Regler mit Regelfehler Begrenzung Initial: k = 0.1, limiit = +/- 100 Sampletime 0.01"/1(pwm_out) -> PWM_Band_Motor/1
  Chart/1(z_soll) -> "P-Regler mit Regelfehler Begrenzung Initial: k = 0.1, limiit = +/- 100 Sampletime 0.01"/2("Z_soll ")
  x_ist/1 -> Chart/2(x_ist)
  y_ist/1 -> Chart/3(y_ist)
  z_ist/1 -> Chart/1(z_ist), "P-Regler mit Regelfehler Begrenzung Initial: k = 0.1, limiit = +/- 100 Sampletime 0.01"/1(Z_ist)

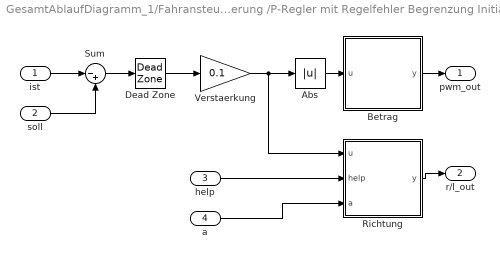
== system GesamtAblaufDiagramm_1/Fahransteuerung /P-Regler mit Regelfehler Begrenzung Initial: k = 0.1, limiit = +//- 100 Sampletime 0.01 ==
  ist : Inport
  soll : Inport  Port=2
  help : Inport  Port=3
  a : Inport  Port=4
  Abs : Abs  SampleTime=0.01
  Betrag : MATLAB Function  TreatAsAtomicUnit=on  SystemSampleTime=0.01
  Dead Zone : DeadZone  LowerValue=-100  UpperValue=100  SampleTime=0.01  SaturateOnIntegerOverflow=on
  Richtung : MATLAB Function  TreatAsAtomicUnit=on  SystemSampleTime=0.01
  Sum : Sum  Inputs=|-+  SampleTime=0.01
  Verstaerkung : Gain  Gain=0.1  SampleTime=0.01
  pwm_out : Outport
  r/l_out : Outport  Port=2
  wires:
  Betrag/1(y) -> pwm_out/1
  Sum/1 -> Dead Zone/1
  Verstaerkung/1 -> Abs/1, Richtung/1(u)
  Dead Zone/1 -> Verstaerkung/1
  Abs/1 -> Betrag/1(u)
  soll/1 -> Sum/2
  Richtung/1(y) -> r/l_out/1
  ist/1 -> Sum/1
  help/1 -> Richtung/2(help)
  a/1 -> Richtung/3(a)

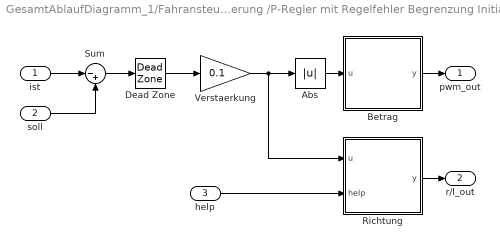
== system GesamtAblaufDiagramm_1/Fahransteuerung /P-Regler mit Regelfehler Begrenzung Initial: k = 0.1, limiit = +//- 100 Sampletime 0.1 ==
  ist : Inport
  soll : Inport  Port=2
  help : Inport  Port=3
  Abs : Abs  SampleTime=0.01
  Betrag : MATLAB Function  TreatAsAtomicUnit=on  SystemSampleTime=0.01
  Dead Zone : DeadZone  LowerValue=-100  UpperValue=100  SampleTime=0.01  SaturateOnIntegerOverflow=on
  Richtung : MATLAB Function  TreatAsAtomicUnit=on  SystemSampleTime=0.01
  Sum : Sum  Inputs=|-+  SampleTime=0.01
  Verstaerkung : Gain  Gain=0.1  SampleTime=0.01
  pwm_out : Outport
  r/l_out : Outport  Port=2
  wires:
  Betrag/1(y) -> pwm_out/1
  Sum/1 -> Dead Zone/1
  Verstaerkung/1 -> Abs/1, Richtung/1(u)
  Dead Zone/1 -> Verstaerkung/1
  Abs/1 -> Betrag/1(u)
  soll/1 -> Sum/2
  Richtung/1(y) -> r/l_out/1
  ist/1 -> Sum/1
  help/1 -> Richtung/2(help)

== system GesamtAblaufDiagramm_1/Modul Positionswerte Sampletime = 0.001 s/Enabled Subsystem ==
  Enable : EnablePort  StatesWhenEnabling=reset
  I2C Receive : c280xlib/I2C Receive  addrFormat=7-Bit addressing  saSource=Specify via dialog  SAR=80  bitCount=8  dataLength=10  initValue=0  NACK=on  STP=off  STR=on  sampleTime=0.001  dataType=uint8
  I2C_Read_Data : Outport
  I2C_Status_Register : Outport  Port=2
  wires:
  I2C Receive/2 -> I2C_Status_Register/1
  I2C Receive/1 -> I2C_Read_Data/1

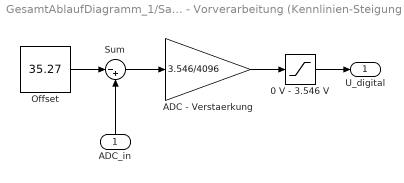
== system GesamtAblaufDiagramm_1/Sammeln/ADC - Messwerte - Vorverarbeitung (Kennlinien-Steigung und Offset-Kompensation) U_digital = (ADC_in - Offset) * 3.546 V // 4096 mit U_digital_max = 3.546 V U_digital_min = 0 V1 ==
  ADC_in : Inport
  0 V - 3.546 V : Saturate  UpperLimit=3.546  LowerLimit=0
  ADC - Verstaerkung : Gain  Gain=3.546/4096
  Offset : Constant  Value=35.27
  Sum : Sum  Inputs=|-+
  U_digital : Outport
  wires:
  ADC_in/1 -> Sum/2
  0 V - 3.546 V/1 -> U_digital/1
  Offset/1 -> Sum/1
  Sum/1 -> ADC - Verstaerkung/1
  ADC - Verstaerkung/1 -> 0 V - 3.546 V/1

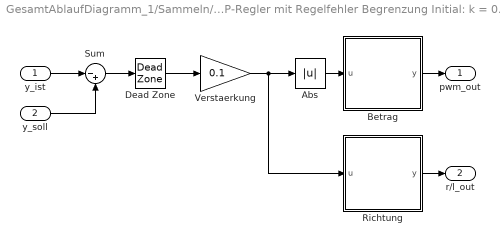
== system GesamtAblaufDiagramm_1/Sammeln/P-Regler mit Regelfehler Begrenzung Initial: k = 0.1, limiit = +//- 100 Sampletime 0.1 ==
  y_ist : Inport
  y_soll : Inport  Port=2
  Abs : Abs  SampleTime=0.01
  Betrag : MATLAB Function  TreatAsAtomicUnit=on  SystemSampleTime=0.01
  Dead Zone : DeadZone  LowerValue=-5  UpperValue=5  SampleTime=0.01  SaturateOnIntegerOverflow=on
  Richtung : MATLAB Function  TreatAsAtomicUnit=on  SystemSampleTime=0.01
  Sum : Sum  Inputs=|-+  SampleTime=0.01
  Verstaerkung : Gain  Gain=0.1  SampleTime=0.01
  pwm_out : Outport
  r/l_out : Outport  Port=2
  wires:
  y_ist/1 -> Sum/1
  Richtung/1(y) -> r/l_out/1
  y_soll/1 -> Sum/2
  Abs/1 -> Betrag/1(u)
  Dead Zone/1 -> Verstaerkung/1
  Verstaerkung/1 -> Richtung/1(u), Abs/1
  Sum/1 -> Dead Zone/1
  Betrag/1(y) -> pwm_out/1

== system GesamtAblaufDiagramm_1/Sortieren/ADC - Messwerte - Vorverarbeitung (Kennlinien-Steigung und Offset-Kompensation) U_digital = (ADC_in - Offset) * 3.546 V // 4096 mit U_digital_max = 3.546 V U_digital_min = 0 V ==
  ADC_in : Inport
  0 V - 3.546 V : Saturate  UpperLimit=3.546  LowerLimit=0
  ADC - Verstaerkung : Gain  Gain=3.546/4096
  Offset : Constant  Value=35.27
  Sum : Sum  Inputs=|-+
  U_digital : Outport
  wires:
  ADC - Verstaerkung/1 -> 0 V - 3.546 V/1
  Sum/1 -> ADC - Verstaerkung/1
  Offset/1 -> Sum/1
  0 V - 3.546 V/1 -> U_digital/1
  ADC_in/1 -> Sum/2

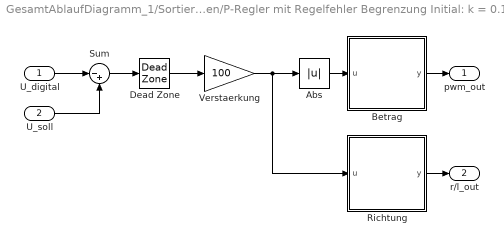
== system GesamtAblaufDiagramm_1/Sortieren/P-Regler mit Regelfehler Begrenzung Initial: k = 0.1, limiit = +//- 100 Sampletime 0.01 ==
  U_digital : Inport
  U_soll : Inport  Port=2
  Abs : Abs  SampleTime=0.01
  Betrag : MATLAB Function  TreatAsAtomicUnit=on  SystemSampleTime=0.01
  Dead Zone : DeadZone  LowerValue=-5  UpperValue=5  SampleTime=0.01  SaturateOnIntegerOverflow=on
  Richtung : MATLAB Function  TreatAsAtomicUnit=on  SystemSampleTime=0.01
  Sum : Sum  Inputs=|-+  SampleTime=0.01
  Verstaerkung : Gain  Gain=100  SampleTime=0.01
  pwm_out : Outport
  r/l_out : Outport  Port=2
  wires:
  Betrag/1(y) -> pwm_out/1
  Sum/1 -> Dead Zone/1
  Verstaerkung/1 -> Abs/1, Richtung/1(u)
  Dead Zone/1 -> Verstaerkung/1
  Abs/1 -> Betrag/1(u)
  U_soll/1 -> Sum/2
  Richtung/1(y) -> r/l_out/1
  U_digital/1 -> Sum/1

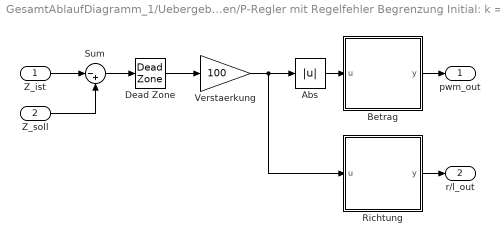
== system GesamtAblaufDiagramm_1/Uebergeben/P-Regler mit Regelfehler Begrenzung Initial: k = 0.1, limiit = +//- 100 Sampletime 0.01 ==
  Z_ist : Inport
  "Z_soll " : Inport  Port=2
  Abs : Abs  SampleTime=0.01
  Betrag : MATLAB Function  TreatAsAtomicUnit=on  SystemSampleTime=0.01
  Dead Zone : DeadZone  LowerValue=-5  UpperValue=5  SampleTime=0.01  SaturateOnIntegerOverflow=on
  Richtung : MATLAB Function  TreatAsAtomicUnit=on  SystemSampleTime=0.01
  Sum : Sum  Inputs=|-+  SampleTime=0.01
  Verstaerkung : Gain  Gain=100  SampleTime=0.01
  pwm_out : Outport
  r/l_out : Outport  Port=2
  wires:
  Betrag/1(y) -> pwm_out/1
  Sum/1 -> Dead Zone/1
  Verstaerkung/1 -> Abs/1, Richtung/1(u)
  Dead Zone/1 -> Verstaerkung/1
  Abs/1 -> Betrag/1(u)
  "Z_soll "/1 -> Sum/2
  Richtung/1(y) -> r/l_out/1
  Z_ist/1 -> Sum/1

== stateflow chart GesamtAblaufDiagramm_1/Modul Positionswerte Sampletime = 0.001 s/Chart1 ==
  state Daten_einlesen
  state x0
  state x1_1
    int16z_bin[0] = int8z_1[0];
    int16z_bin[1] = int8z_1[1];
    int16z_bin[2] = int8z_1[2];
    int16z_bin[3] = int8z_1[3];
    int16z_bin[4] = int8z_1[4];
    int16z_bin[5] = int8z_1[5]
    int16z_bin[6] = int8z_1[6];
    int16z_bin[7] = int8z_1[7];
    int16z_bin[8] = int8z_2[0];
    int16z_bin[9] = int8z_2[1];
    int16z_bin[10] = int8z_2[2];
    int16z_bin[11] = int8z_2[3];
    int16z_bin[12] = int8z_2[4];
    int16z_bin[13] = int8z_2[5]
    int16z_bin[14] = int8z_2[6];
    int16z_bin[15] = int8z_2[7];
  x0 -> Daten_einlesen
  (default) -> x0
  Daten_einlesen -> x1_1
  x1_1 -> Daten_einlesen
  data: int8z_1 input size=8; int8z_2 input size=8; int16z_bin output size=16 =0

== stateflow chart GesamtAblaufDiagramm_1/Uebergeben/Chart ==
  state Start
  state Laufen_Hoch
    entry:z_soll=500;
  state Stop
    entry:z_soll=z_ist;
  state Stop
    entry:z_soll=z_ist;
  state Laufen_rueck
    entry:z_soll=10;
  (default) -> Start
  Start -> Laufen_Hoch : [y_ist<405&&y_ist>395&&x_ist<1105&&x_ist>1095]
  Laufen_rueck -> Stop : [z_ist<15&&z_ist>5]
  Laufen_Hoch -> Stop : [z_ist<505&&z_ist>495]
  Stop -> Laufen_rueck : [after(2,sec)]
  data: z_ist input; z_soll output double; x_ist input; y_ist input

== stateflow chart GesamtAblaufDiagramm_1/Modul Positionswerte Sampletime = 0.001 s/Chart2 ==
  state Daten_einlesen
  state x0
  state x1_1
    int16y_bin[0] = int8y_1[0];
    int16y_bin[1] = int8y_1[1];
    int16y_bin[2] = int8y_1[2];
    int16y_bin[3] = int8y_1[3];
    int16y_bin[4] = int8y_1[4];
    int16y_bin[5] = int8y_1[5]
    int16y_bin[6] = int8y_1[6];
    int16y_bin[7] = int8y_1[7];
    int16y_bin[8] = int8y_2[0];
    int16y_bin[9] = int8y_2[1];
    int16y_bin[10] = int8y_2[2];
    int16y_bin[11] = int8y_2[3];
    int16y_bin[12] = int8y_2[4];
    int16y_bin[13] = int8y_2[5]
    int16y_bin[14] = int8y_2[6];
    int16y_bin[15] = int8y_2[7];
  x0 -> Daten_einlesen
  (default) -> x0
  Daten_einlesen -> x1_1
  x1_1 -> Daten_einlesen
  data: int8y_1 input size=8; int8y_2 input size=8; int16y_bin output size=16 =0

== matlab function GesamtAblaufDiagramm_1/Uebergeben/P-Regler mit Regelfehler Begrenzung Initial: k = 0.1, limiit = +//- 100 Sampletime 0.01/Betrag ==
  settings: updateMethod=DISCRETE  sampleTime=0.01
  data: u input; y output
function y = fcn( u )

if 0.5 < u && u < 60
    y = 60;
elseif u <= 0.5
    y = 0;
elseif u >= 100
    y = 100;
else
    y = abs(u);
end

== stateflow chart GesamtAblaufDiagramm_1/Modul Positionswerte Sampletime = 0.001 s/Chart4 ==
  state Daten_einlesen
  state x0
  state x1_1
    int16a1_bin[0] = int8a1_1[0];
    int16a1_bin[1] = int8a1_1[1];
    int16a1_bin[2] = int8a1_1[2];
    int16a1_bin[3] = int8a1_1[3];
    int16a1_bin[4] = int8a1_1[4];
    int16a1_bin[5] = int8a1_1[5]
    int16a1_bin[6] = int8a1_1[6];
    int16a1_bin[7] = int8a1_1[7];
    int16a1_bin[8] = int8a1_2[0];
    int16a1_bin[9] = int8a1_2[1];
    int16a1_bin[10] = int8a1_2[2];
    int16a1_bin[11] = int8a1_2[3];
    int16a1_bin[12] = int8a1_2[4];
    int16a1_bin[13] = int8a1_2[5]
    int16a1_bin[14] = int8a1_2[6];
    int16a1_bin[15] = int8a1_2[7];
  x0 -> Daten_einlesen
  (default) -> x0
  Daten_einlesen -> x1_1
  x1_1 -> Daten_einlesen
  data: int8a1_1 input size=8; int8a1_2 input size=8; int16a1_bin output size=16 =0

== matlab function GesamtAblaufDiagramm_1/Uebergeben/P-Regler mit Regelfehler Begrenzung Initial: k = 0.1, limiit = +//- 100 Sampletime 0.01/Richtung ==
  settings: updateMethod=DISCRETE  sampleTime=0.01
  data: u input; y output
function y = fcn( u )

if u > 0
    y = 1;
else
    y = 0;
end

== stateflow chart GesamtAblaufDiagramm_1/Modul Positionswerte Sampletime = 0.001 s/Chart6 ==
  state Daten_einlesen
  state x0
  state x1_1
    int16x_bin[0] = int8x_1[0];
    int16x_bin[1] = int8x_1[1];
    int16x_bin[2] = int8x_1[2];
    int16x_bin[3] = int8x_1[3];
    int16x_bin[4] = int8x_1[4];
    int16x_bin[5] = int8x_1[5]
    int16x_bin[6] = int8x_1[6];
    int16x_bin[7] = int8x_1[7];
    int16x_bin[8] = int8x_2[0];
    int16x_bin[9] = int8x_2[1];
    int16x_bin[10] = int8x_2[2];
    int16x_bin[11] = int8x_2[3];
    int16x_bin[12] = int8x_2[4];
    int16x_bin[13] = int8x_2[5]
    int16x_bin[14] = int8x_2[6];
    int16x_bin[15] = int8x_2[7];
  x0 -> Daten_einlesen
  (default) -> x0
  Daten_einlesen -> x1_1
  x1_1 -> Daten_einlesen
  data: int8x_1 input size=8; int8x_2 input size=8; int16x_bin output size=16 =0

== stateflow chart GesamtAblaufDiagramm_1/Sortieren/Sortieren ==
  state Start
  state Sammeln_Blau
    U_soll=170
  state Sammeln_RotUndSchwarz
    entry:U_soll=190
  state Reset_B
    state Stop
      entry:U_digital=U_soll;
    state Ruecklaufen
      entry:U_soll=190;
    (default) -> Reset_B.Stop
    Reset_B.Stop -> Reset_B.Ruecklaufen
  state Reset_R_S
    state Stop
      entry:U_digital=U_soll;
    state Ruecklaufen
      entry:U_sol=170;
    (default) -> Reset_R_S.Stop
    Reset_R_S.Stop -> Reset_R_S.Ruecklaufen
  (default) -> Start
  Sammeln_RotUndSchwarz -> ? : [after(1,sec)]
  Start -> Sammeln_Blau [order 1] : [U_digital>1.8]
  Reset_B -> Start : [after(1,sec)]
  Reset_R_S -> Start : [after(1,sec)]
  Start -> Sammeln_RotUndSchwarz [order 2] : [U_digital<1.8]
  Sammeln_Blau -> Reset_B : [after(1,sec)]
  data: U_digital input; U_soll output double

== stateflow chart GesamtAblaufDiagramm_1/Modul Positionswerte Sampletime = 0.001 s/Chart8 ==
  state init
    values_out1[0] = 0;
    values_out1[1] = 0;
    values_out1[2] = 0;
    values_out1[3] = 0;
    values_out1[4] = 0;
    values_out1[5] = 0;
    values_out1[6] = 0;
    values_out1[7] = 0;
    values_out1[8] = 0;
    values_out1[9] = 0;
    values_out1[10] = 0;
    values_out1[11] = 0;
    values_out1[12] = 0;
    values_out1[13] = 0;
    values_out1[14] = 0;
    values_out1[15] = 0;
    values_out1[16] = 0;
    values_out1[17] = 0;
    values_out1[18] = 0;
    values_out1[19] = 0;
  state wert_erkannt
    values_out1[0] = in_data[0];
    values_out1[1] = in_data[1];
    values_out1[2] = in_data[2];
    values_out1[3] = in_data[3];
    values_out1[4] = in_data[4];
    values_out1[5] = in_data[5];
    values_out1[6] = in_data[6];
    values_out1[7] = in_data[7];
    values_out1[8] = in_data[8];
    values_out1[9] = in_data[9];
  state Anfang_found_Schritt_uebertragen_weglassen_performance
    x_found = x_found +1;
  state x5_valid_data_found1
    valid_values1 = values_out1[search+1];
    valid_values2 = values_out1[search+2];
    valid_values3 = values_out1[search+3];
    valid_values4 = values_out1[search+4];
    valid_values5 = values_out1[search+5];
    valid_values6 = values_out1[search+6];
    valid_values7 = values_out1[search+7];
    valid_values8 = values_out1[search+8];
    zaehler = zaehler +1;
  state wert_erkannt2
    values_out1[10] = in_data[0];
    values_out1[11] = in_data[1];
    values_out1[12] = in_data[2];
    values_out1[13] = in_data[3];
    values_out1[14] = in_data[4];
    values_out1[15] = in_data[5];
    values_out1[16] = in_data[6];
    values_out1[17] = in_data[7];
    values_out1[18] = in_data[8];
    values_out1[19] = in_data[9];
    search = 0;
    counter = counter + 1;
  state x1_search1
    search = search + 1;
  x5_valid_data_found1 -> wert_erkannt
  x1_search1 -> wert_erkannt [order 3]
  init -> wert_erkannt
  (default) -> init
  Anfang_found_Schritt_uebertragen_weglassen_performance -> x5_valid_data_found1 [order 1] : [((values_out1[search]+values_out1[search+1]+values_out1[search+2]+values_out1[search+3]+values_out1[search+4]+values_out1[search+5]+values_out1[search+6]+values_out1[search+7]+values_out1[search+8])) == values_out1[search+9]]
  wert_erkannt -> wert_erkannt2
  Anfang_found_Schritt_uebertragen_weglassen_performance -> x5_valid_data_found1 [order 2] : [((values_out1[search]+values_out1[search+1]+values_out1[search+2]+values_out1[search+3]+values_out1[search+4]+values_out1[search+5]+values_out1[search+6]+values_out1[search+7]+values_out1[search+8])-(256)) == values_out1[search+9]]
  Anfang_found_Schritt_uebertragen_weglassen_performance -> x5_valid_data_found1 [order 3] : [((values_out1[search]+values_out1[search+1]+values_out1[search+2]+values_out1[search+3]+values_out1[search+4]+values_out1[search+5]+values_out1[search+6]+values_out1[search+7]+values_out1[search+8])-(512)) == values_out1[search+9]]
  Anfang_found_Schritt_uebertragen_weglassen_performance -> x5_valid_data_found1 [order 7] : [((values_out1[search]+values_out1[search+1]+values_out1[search+2]+values_out1[search+3]+values_out1[search+4]+values_out1[search+5]+values_out1[search+6]+values_out1[search+7]+values_out1[search+8])-(768)) == values_out1[search+9]]
  Anfang_found_Schritt_uebertragen_weglassen_performance -> x5_valid_data_found1 [order 6] : [((values_out1[search]+values_out1[search+1]+values_out1[search+2]+values_out1[search+3]+values_out1[search+4]+values_out1[search+5]+values_out1[search+6]+values_out1[search+7]+values_out1[search+8])-(1024)) == values_out1[search+9]]
  Anfang_found_Schritt_uebertragen_weglassen_performance -> x5_valid_data_found1 [order 5] : [((values_out1[search]+values_out1[search+1]+values_out1[search+2]+values_out1[search+3]+values_out1[search+4]+values_out1[search+5]+values_out1[search+6]+values_out1[search+7]+values_out1[search+8])-(1280)) == values_out1[search+9]]
  Anfang_found_Schritt_uebertragen_weglassen_performance -> x5_valid_data_found1 [order 4] : [((values_out1[search]+values_out1[search+1]+values_out1[search+2]+values_out1[search+3]+values_out1[search+4]+values_out1[search+5]+values_out1[search+6]+values_out1[search+7]+values_out1[search+8])-(1536)) == values_out1[search+9]]
  Anfang_found_Schritt_uebertragen_weglassen_performance -> x5_valid_data_found1 [order 8] : [((values_out1[search]+values_out1[search+1]+values_out1[search+2]+values_out1[search+3]+values_out1[search+4]+values_out1[search+5]+values_out1[search+6]+values_out1[search+7]+values_out1[search+8])-(1792)) == values_out1[search+9]]
  Anfang_found_Schritt_uebertragen_weglassen_performance -> x5_valid_data_found1 [order 10] : [((values_out1[search]+values_out1[search+1]+values_out1[search+2]+values_out1[search+3]+values_out1[search+4]+values_out1[search+5]+values_out1[search+6]+values_out1[search+7]+values_out1[search+8])-(2048)) == values_out1[search+9]]
  Anfang_found_Schritt_uebertragen_weglassen_performance -> x1_search1 [order 9]
  wert_erkannt2 -> Anfang_found_Schritt_uebertragen_weglassen_performance [order 1] : [values_out1[search] == 88]
  x1_search1 -> Anfang_found_Schritt_uebertragen_weglassen_performance [order 1] : [values_out1[search] == 88]
  wert_erkannt2 -> x1_search1 [order 2]
  x1_search1 -> x1_search1 [order 2] : [search < 19]
  data: in_data input size=10; values_out1 local int16 size=20; zaehler local int32 =0; search local int16; valid_values1 output int16 size=1; valid_values2 output int16 size=1; valid_values3 output int16 size=1; valid_values4 output int16 size=1; valid_values5 output int16 size=1; valid_values6 output int16 size=1; valid_values7 output int16 size=1; valid_values8 output int16 size=1; counter local int32 =0; x_found local int32 =0

== matlab function GesamtAblaufDiagramm_1/Sortieren/P-Regler mit Regelfehler Begrenzung Initial: k = 0.1, limiit = +//- 100 Sampletime 0.01/Betrag ==
  settings: updateMethod=DISCRETE  sampleTime=0.01
  data: u input; y output
function y = fcn( u )

if 0.5 < u && u < 60
    y = 60;
elseif u <= 0.5
    y = 0;
elseif u >= 100
    y = 100;
else
    y = abs(u);
end
